simulink model "testHeatPumpBasic"  (R2013b)
settings: Solver=ode45  StartTime=0.0  StopTime=1*24*3600  RelTol=1e-4  AbsTol=1e-5
libraries: carnot x5
settings Model: Creator=drhf  LastModifiedBy=drhf
settings OptimizationCC: ExpressionDepthLimit=2147483647
settings DebuggingCC: StateNameClashWarn=warning
settings GRTTargetCC: CombineOutputUpdateFcns=off  GRTInterface=on

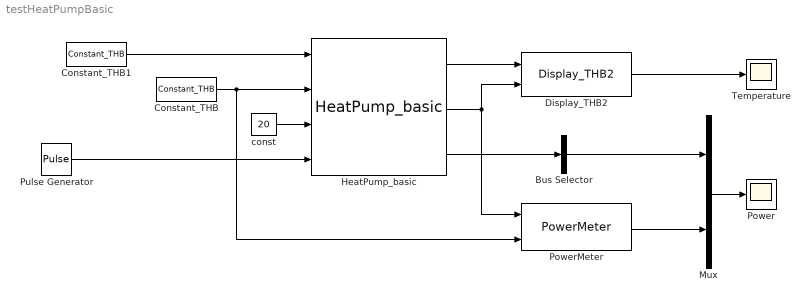
== system testHeatPumpBasic ==
  Bus Selector : BusSelector  OutputSignals=Pelec,Qdot_cold,Qdot_hot  OutputAsBus=on
  Constant_THB : carnot/Source/Simple/Constant_THB  t=40  mdot=2000/3600  p=1e5  mID=No Pressure Drop  fluid=Water  mix=0  mix2=0  mix3=0  dia=0.02  hgt=0
  Constant_THB1 : carnot/Source/Simple/Constant_THB  t=5  mdot=2000/3600  p=1e5  mID=No Pressure Drop  fluid=Water  mix=0  mix2=0  mix3=0  dia=0.02  hgt=0
  Display_THB2 : carnot/Outputs/Display_THB2  t=on  m=off  p=off  id=off  mix=off  d=off
  HeatPump_basic : carnot/Basic/Thermal_Models/HeatPump_basic  K="[300 -60 1250  -6.67   60   -5.13e-5   306.7   -115 12225]"  caph=5*4182  capc=5*4182  UA=1
  Mux : Mux  Inputs=2
  Power : Scope
      settings: TickLabels=on  YMin=-20000  YMax=20000
  PowerMeter : carnot/Control/PowerMeter
  Pulse Generator : DiscretePulseGenerator  PulseType=Time based  Period=3600  PulseWidth=50
  Temperature : Scope
      settings: TickLabels=on  YMin=-20  YMax=50
  const : Constant  Value=20
  wires:
  Pulse Generator/1 -> HeatPump_basic/4
  Display_THB2/1 -> Temperature/1
  Mux/1 -> Power/1
  PowerMeter/1 -> Mux/2
  Bus Selector/1 -> Mux/1
  HeatPump_basic/3 -> Bus Selector/1
  HeatPump_basic/1 -> Display_THB2/1
  HeatPump_basic/2 -> Display_THB2/2, PowerMeter/1
  const/1 -> HeatPump_basic/3
  Constant_THB/1 -> HeatPump_basic/2, PowerMeter/2
  Constant_THB1/1 -> HeatPump_basic/1
